simulink model "Step_Test"  (R2017b)
settings: Solver=VariableStepAuto  StartTime=0.0  StopTime=500  RelTol=1e-3  EnableMultiTasking=on
StartFcn:
  | clear all
libraries: realtime_pacer_lib x1
settings Model: Creator=johnh  LastModifiedBy=johnh
settings OptimizationCC: LifeSpan=inf
settings DebuggingCC: SFUnexpectedBacktrackingDiag=warning  SFNoUnconditionalDefaultTransitionDiag=warning  SFExecutionAtInitializationDiag=none
settings CodeAppCC: StateflowObjectComments=on
settings GRTTargetCC: TargetLangStandard=C89/C90 (ANSI)  GeneratePreprocessorConditionals=Disable all
settings ConfigComp: CovMetricSettings=dw  CovHtmlReporting=on  CovSaveCumulativeToWorkspaceVar=on  CovSaveSingleToWorkspaceVar=on  CovExternalEMLEnable=off

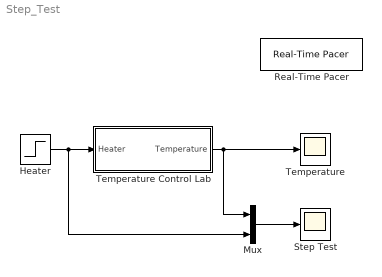
== system Step_Test ==
  Heater : Step  Time=10  After=80  SampleTime=0
  Mux : Mux  Inputs=2
  Real-Time Pacer : realtime_pacer_lib/Real-Time Pacer  simTimePerRealTime=1
  Step Test : Scope
  Temperature : Scope
  Temperature Control Lab : Subsystem
  wires:
  Heater/1 -> Mux/2, Temperature Control Lab/1(Heater)
  Temperature Control Lab/1(Temperature) -> Mux/1, Temperature/1
  Mux/1 -> Step Test/1

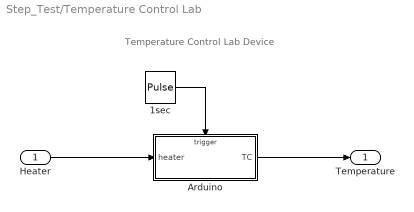
== system Step_Test/Temperature Control Lab ==
  note: Temperature Control Lab Device
  Heater : Inport
  1sec : DiscretePulseGenerator  PulseType=Time based  Period=1  PulseWidth=50
  Arduino : Subsystem  TreatAsAtomicUnit=on
  Temperature : Outport
  wires:
  1sec/1 -> Arduino/Trigger
  Arduino/1(TC) -> Temperature/1
  Heater/1 -> Arduino/1(heater)

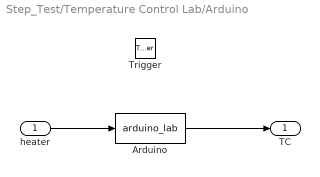
== system Step_Test/Temperature Control Lab/Arduino ==
  heater : Inport
  Trigger : TriggerPort  VariantControl=Variant
  Arduino : MATLABFcn  MATLABFcn=arduino_lab
  TC : Outport  InitialOutput=23
  wires:
  heater/1 -> Arduino/1
  Arduino/1 -> TC/1
